simulink model "rectangle_method_R2018b"  (R2018b)
settings: Solver=VariableStepAuto  StartTime=0.0  StopTime=2  MaxStep=0.001  RelTol=1e-3
undefined symbols (not defined in the file): Ki, Kia, T0
settings Model: Creator=Anton Mayorov  LastModifiedBy=bedla
settings SFSimCC: SimUseLocalCustomCode=off
settings RTWCC: RTWUseLocalCustomCode=off

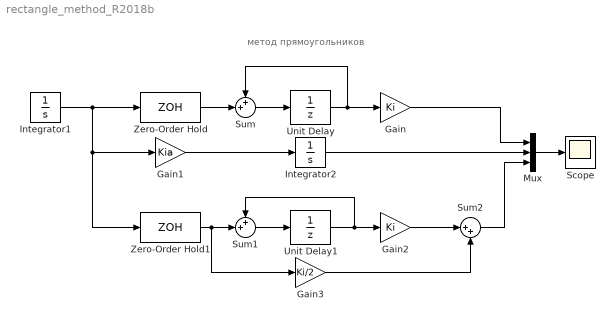
== system rectangle_method_R2018b ==
  note: метод прямоугольников
  Gain : Gain  Gain=Ki
  Gain1 : Gain  Gain=Kia
  Gain2 : Gain  Gain=Ki
  Gain3 : Gain  Gain=Ki/2
  Integrator1 : Integrator  InitialCondition=1
  Integrator2 : Integrator
  Mux : Mux  Inputs=3
  Scope : Scope
  Sum : Sum  Inputs=++|
  Sum1 : Sum  Inputs=++|
  Sum2 : Sum  Inputs=|++
  Unit Delay : UnitDelay  SampleTime=-1  HasFrameUpgradeWarning=on
  Unit Delay1 : UnitDelay  SampleTime=-1  HasFrameUpgradeWarning=on
  Zero-Order Hold : ZeroOrderHold  SampleTime=T0
  Zero-Order Hold1 : ZeroOrderHold  SampleTime=T0
  wires:
  Mux/1 -> Scope/1
  Gain1/1 -> Integrator2/1
  Integrator2/1 -> Mux/2
  Zero-Order Hold/1 -> Sum/2
  Unit Delay/1 -> Sum/1, Gain/1
  Sum/1 -> Unit Delay/1
  Gain/1 -> Mux/1
  Gain2/1 -> Sum2/1
  Integrator1/1 -> Gain1/1, Zero-Order Hold1/1, Zero-Order Hold/1
  Zero-Order Hold1/1 -> Sum1/2, Gain3/1
  Sum1/1 -> Unit Delay1/1
  Unit Delay1/1 -> Gain2/1, Sum1/1
  Gain3/1 -> Sum2/2
  Sum2/1 -> Mux/3
